simulink subsystem "MulticopterScheduler"  (R2023b)
settings: Solver=VariableStepAuto  StartTime=0.0  StopTime=10.0  RelTol=1e-3
undefined symbols (not defined in the file): CriticalTiltAngle, DiscIntNeverNeededParam, FWTrimSpeed, tilt_max, tilt_trim, uavParam, w_trim, WindDownRate
settings Model: Creator=The MathWorks, Inc.  LastModifiedBy=The MathWorks, Inc.

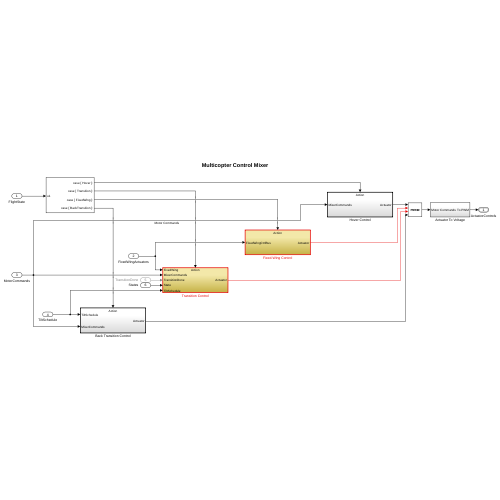
[thumbnail: Simulink's stored preview of the top-level diagram]
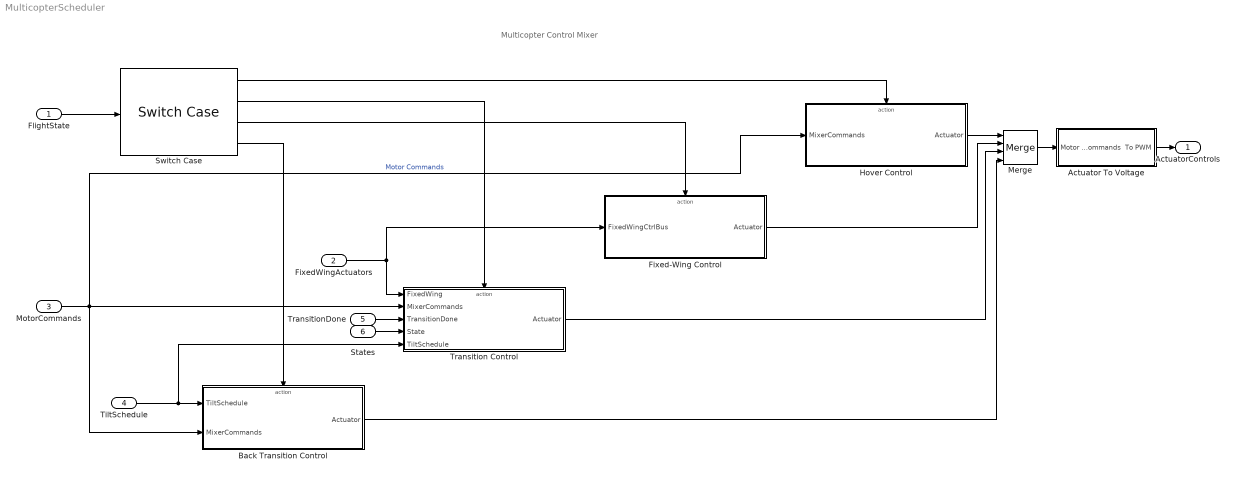
== system MulticopterScheduler ==
  note: Multicopter Control Mixer
  FlightState : Inport
  FixedWingActuators : Inport  Port=2
  MotorCommands : Inport  Port=3
  TiltSchedule : Inport  Port=4
  TransitionDone : Inport  Port=5
  States : Inport  Port=6
  Actuator To Voltage : Subsystem
  Back Transition Control : Subsystem  TreatAsAtomicUnit=on
  Fixed-Wing Control : Subsystem  TreatAsAtomicUnit=on
  Hover Control : Subsystem  TreatAsAtomicUnit=on
  Merge : Merge  Inputs=4
  Switch Case : SwitchCase  CaseConditions={flightState.Hover, flightState.Transition, flightState.FixedWing, flightState.BackTransition}  ShowDefaultCase=off
  Transition Control : Subsystem  TreatAsAtomicUnit=on
  ActuatorControls : Outport  OutDataTypeStr=Bus: RotorCntrlBus
  wires:
  Fixed-Wing Control/1(Actuator) -> Merge/2
  TiltSchedule/1 -> Transition Control/5(TiltSchedule), Back Transition Control/1(TiltSchedule)
  Switch Case/1 -> Hover Control/Action
  Merge/1 -> Actuator To Voltage/1(Motor Commands)
  FixedWingActuators/1 -> Transition Control/1(FixedWing), Fixed-Wing Control/1(FixedWingCtrlBus)
  Hover Control/1(Actuator) -> Merge/1
  Transition Control/1(Actuator) -> Merge/3
  FlightState/1 -> Switch Case/1
  TransitionDone/1 -> Transition Control/3(TransitionDone)
  States/1 -> Transition Control/4(State)
  Switch Case/4 -> Back Transition Control/Action
  Back Transition Control/1(Actuator) -> Merge/4
  MotorCommands/1 -> Back Transition Control/2(MixerCommands), Transition Control/2(MixerCommands), Hover Control/1(MixerCommands)  "Motor Commands"
  Actuator To Voltage/1(To PWM) -> ActuatorControls/1
  Switch Case/3 -> Fixed-Wing Control/Action
  Switch Case/2 -> Transition Control/Action

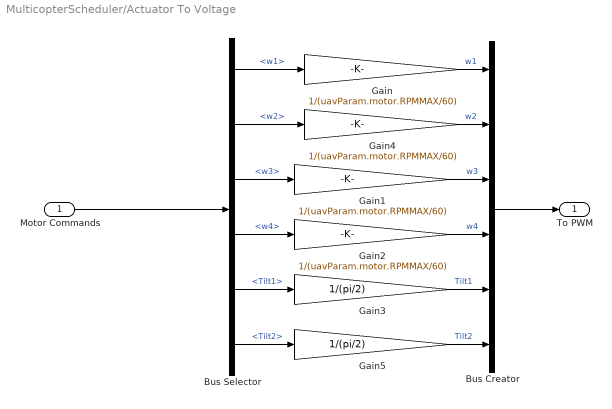
== system MulticopterScheduler/Actuator To Voltage ==
  Motor Commands : Inport
  Bus Creator : BusCreator  Inputs=6  OutDataTypeStr=Bus: RotorCntrlBus
  Bus Selector : BusSelector  OutputSignals=w1,w2,w3,w4,Tilt1,Tilt2
  Gain{,1..2,4} (4 alike) : Gain  Gain=1/(uavParam.motor.RPMMAX/60)
  Gain3 : Gain  Gain=1/(pi/2)
  Gain5 : Gain  Gain=1/(pi/2)
  To PWM : Outport
  wires:
  Bus Creator/1 -> To PWM/1
  Gain5/1 -> Bus Creator/6  "Tilt2"
  Gain3/1 -> Bus Creator/5  "Tilt1"
  Gain2/1 -> Bus Creator/4  "w4"
  Gain1/1 -> Bus Creator/3  "w3"
  Gain4/1 -> Bus Creator/2  "w2"
  Gain/1 -> Bus Creator/1  "w1"
  Bus Selector/6 -> Gain5/1  "<Tilt2>"
  Bus Selector/5 -> Gain3/1  "<Tilt1>"
  Bus Selector/4 -> Gain2/1  "<w4>"
  Bus Selector/2 -> Gain4/1  "<w2>"
  Bus Selector/3 -> Gain1/1  "<w3>"
  Bus Selector/1 -> Gain/1  "<w1>"
  Motor Commands/1 -> Bus Selector/1

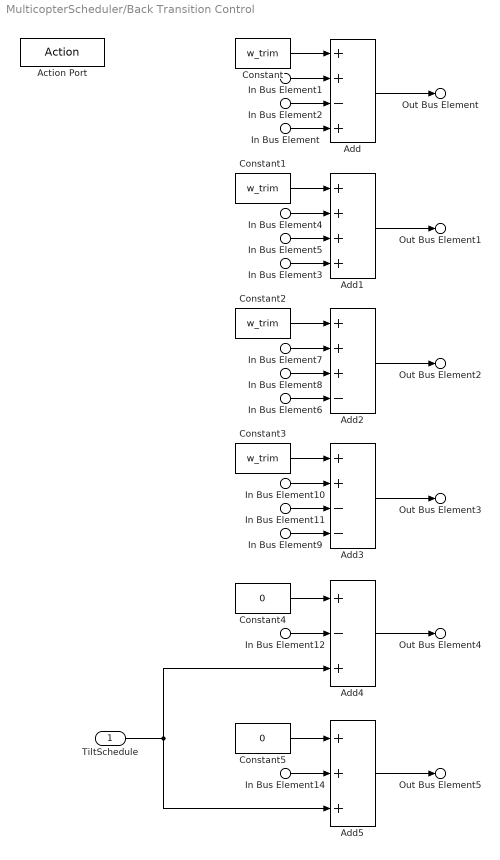
== system MulticopterScheduler/Back Transition Control ==
  TiltSchedule : Inport
  In Bus Element{,3,6,9} (4 alike) : Inport  Port=2  PortName=MixerCommands  Element=w_theta
  In Bus Element{1,4,7,10} (4 alike) : Inport  Port=2  PortName=MixerCommands  Element=w_z
  In Bus Element{2,5,8,11} (4 alike) : Inport  Port=2  PortName=MixerCommands  Element=w_phi
  In Bus Element12 : Inport  Port=2  PortName=MixerCommands  Element=l_psi
  In Bus Element14 : Inport  Port=2  PortName=MixerCommands  Element=l_psi
  Action Port : ActionPort
  Add : Sum  Inputs=++-+
  Add1 : Sum  Inputs=++++
  Add2 : Sum  Inputs=+++-
  Add3 : Sum  Inputs=++--
  Add4 : Sum  Inputs=+-+
  Add5 : Sum  Inputs=+++
  Constant{,1..3} (4 alike) : Constant  Value=w_trim
  Constant4 : Constant  Value=0
  Constant5 : Constant  Value=0
  Out Bus Element : Outport  PortName=Actuator  Element=w1
  Out Bus Element1 : Outport  PortName=Actuator  Element=w2
  Out Bus Element2 : Outport  PortName=Actuator  Element=w3
  Out Bus Element3 : Outport  PortName=Actuator  Element=w4
  Out Bus Element4 : Outport  PortName=Actuator  Element=Tilt1
  Out Bus Element5 : Outport  PortName=Actuator  Element=Tilt2
  wires:
  Add5/1 -> Out Bus Element5/1
  Add4/1 -> Out Bus Element4/1
  In Bus Element14/1 -> Add5/2
  Constant5/1 -> Add5/1
  TiltSchedule/1 -> Add5/3, Add4/3
  In Bus Element12/1 -> Add4/2
  Constant4/1 -> Add4/1
  In Bus Element7/1 -> Add2/2
  Add3/1 -> Out Bus Element3/1
  Add2/1 -> Out Bus Element2/1
  Add/1 -> Out Bus Element/1
  Constant3/1 -> Add3/1
  Constant/1 -> Add/1
  Add1/1 -> Out Bus Element1/1
  In Bus Element1/1 -> Add/2
  In Bus Element10/1 -> Add3/2
  Constant1/1 -> Add1/1
  In Bus Element6/1 -> Add2/4
  In Bus Element9/1 -> Add3/4
  Constant2/1 -> Add2/1
  In Bus Element8/1 -> Add2/3
  In Bus Element11/1 -> Add3/3
  In Bus Element/1 -> Add/4
  In Bus Element3/1 -> Add1/4
  In Bus Element5/1 -> Add1/3
  In Bus Element2/1 -> Add/3
  In Bus Element4/1 -> Add1/2

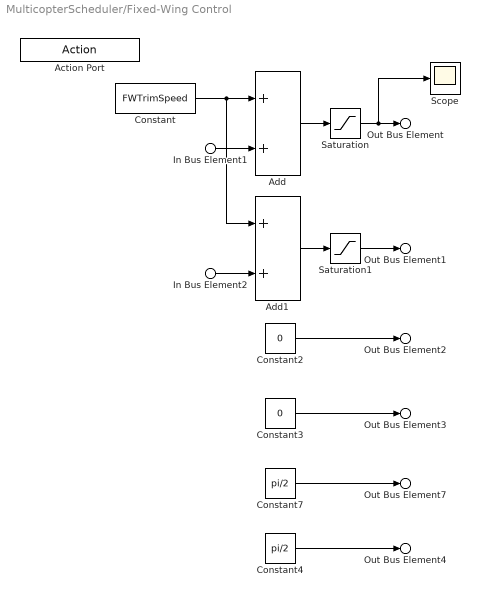
== system MulticopterScheduler/Fixed-Wing Control ==
  In Bus Element2 : Inport  PortName=FixedWingCtrlBus  Element=dT
  In Bus Element1 : Inport  PortName=FixedWingCtrlBus  Element=dT
  Action Port : ActionPort
  Add : Sum
  Add1 : Sum
  Constant : Constant  Value=FWTrimSpeed
  Constant2 : Constant  Value=0
  Constant3 : Constant  Value=0
  Constant4 : Constant  Value=pi/2
  Constant7 : Constant  Value=pi/2
  Saturation : Saturate  UpperLimit=Inf  LowerLimit=0
  Saturation1 : Saturate  UpperLimit=Inf  LowerLimit=0
  Scope : Scope
  Out Bus Element : Outport  PortName=Actuator  Element=w1
  Out Bus Element1 : Outport  PortName=Actuator  Element=w2
  Out Bus Element2 : Outport  PortName=Actuator  Element=w3
  Out Bus Element3 : Outport  PortName=Actuator  Element=w4
  Out Bus Element7 : Outport  PortName=Actuator  Element=Tilt1
  Out Bus Element4 : Outport  PortName=Actuator  Element=Tilt2
  wires:
  Constant3/1 -> Out Bus Element3/1
  Saturation1/1 -> Out Bus Element1/1
  Saturation/1 -> Out Bus Element/1, Scope/1
  In Bus Element1/1 -> Add/2
  Add/1 -> Saturation/1
  In Bus Element2/1 -> Add1/2
  Constant7/1 -> Out Bus Element7/1
  Constant/1 -> Add/1, Add1/1
  Constant2/1 -> Out Bus Element2/1
  Constant4/1 -> Out Bus Element4/1
  Add1/1 -> Saturation1/1

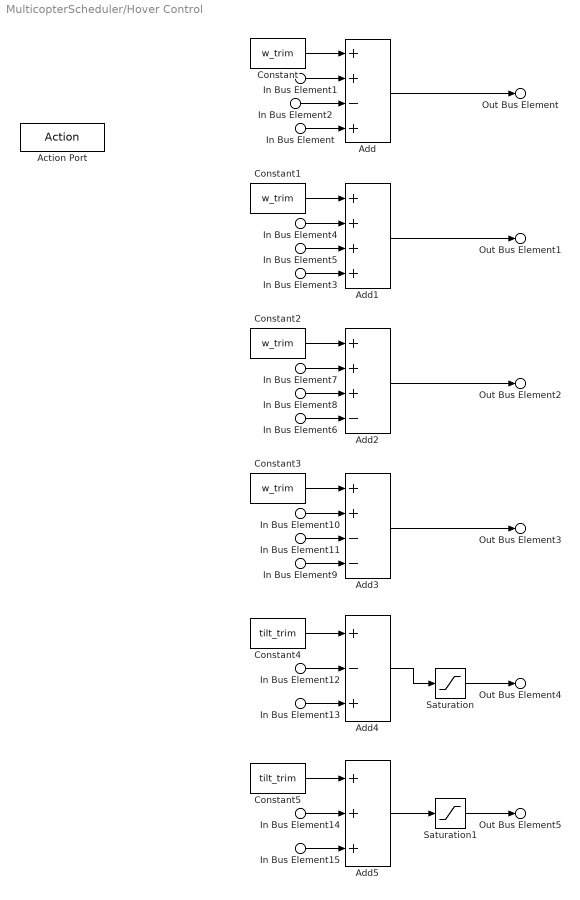
== system MulticopterScheduler/Hover Control ==
  In Bus Element{,3,6,9} (4 alike) : Inport  PortName=MixerCommands  Element=w_theta
  In Bus Element{1,4,7,10} (4 alike) : Inport  PortName=MixerCommands  Element=w_z
  In Bus Element{2,5,8,11} (4 alike) : Inport  PortName=MixerCommands  Element=w_phi
  In Bus Element12 : Inport  PortName=MixerCommands  Element=l_psi
  In Bus Element14 : Inport  PortName=MixerCommands  Element=l_psi
  In Bus Element13 : Inport  PortName=MixerCommands  Element=l_x
  In Bus Element15 : Inport  PortName=MixerCommands  Element=l_x
  Action Port : ActionPort
  Add : Sum  Inputs=++-+
  Add1 : Sum  Inputs=++++
  Add2 : Sum  Inputs=+++-
  Add3 : Sum  Inputs=++--
  Add4 : Sum  Inputs=+-+
  Add5 : Sum  Inputs=+++
  Constant{,1..3} (4 alike) : Constant  Value=w_trim
  Constant4 : Constant  Value=tilt_trim
  Constant5 : Constant  Value=tilt_trim
  Saturation : Saturate  UpperLimit=tilt_max  LowerLimit=-tilt_max
  Saturation1 : Saturate  UpperLimit=tilt_max  LowerLimit=-tilt_max
  Out Bus Element : Outport  PortName=Actuator  Element=w1
  Out Bus Element1 : Outport  PortName=Actuator  Element=w2
  Out Bus Element2 : Outport  PortName=Actuator  Element=w3
  Out Bus Element3 : Outport  PortName=Actuator  Element=w4
  Out Bus Element4 : Outport  PortName=Actuator  Element=Tilt1
  Out Bus Element5 : Outport  PortName=Actuator  Element=Tilt2
  wires:
  In Bus Element15/1 -> Add5/3
  In Bus Element14/1 -> Add5/2
  In Bus Element13/1 -> Add4/3
  In Bus Element12/1 -> Add4/2
  Saturation1/1 -> Out Bus Element5/1
  Saturation/1 -> Out Bus Element4/1
  Add3/1 -> Out Bus Element3/1
  Add2/1 -> Out Bus Element2/1
  Add1/1 -> Out Bus Element1/1
  Add/1 -> Out Bus Element/1
  In Bus Element7/1 -> Add2/2
  Add4/1 -> Saturation/1
  Constant3/1 -> Add3/1
  Constant/1 -> Add/1
  Constant4/1 -> Add4/1
  In Bus Element1/1 -> Add/2
  In Bus Element10/1 -> Add3/2
  Constant1/1 -> Add1/1
  In Bus Element6/1 -> Add2/4
  In Bus Element9/1 -> Add3/4
  Constant2/1 -> Add2/1
  In Bus Element8/1 -> Add2/3
  In Bus Element11/1 -> Add3/3
  In Bus Element/1 -> Add/4
  Add5/1 -> Saturation1/1
  In Bus Element3/1 -> Add1/4
  Constant5/1 -> Add5/1
  In Bus Element5/1 -> Add1/3
  In Bus Element2/1 -> Add/3
  In Bus Element4/1 -> Add1/2

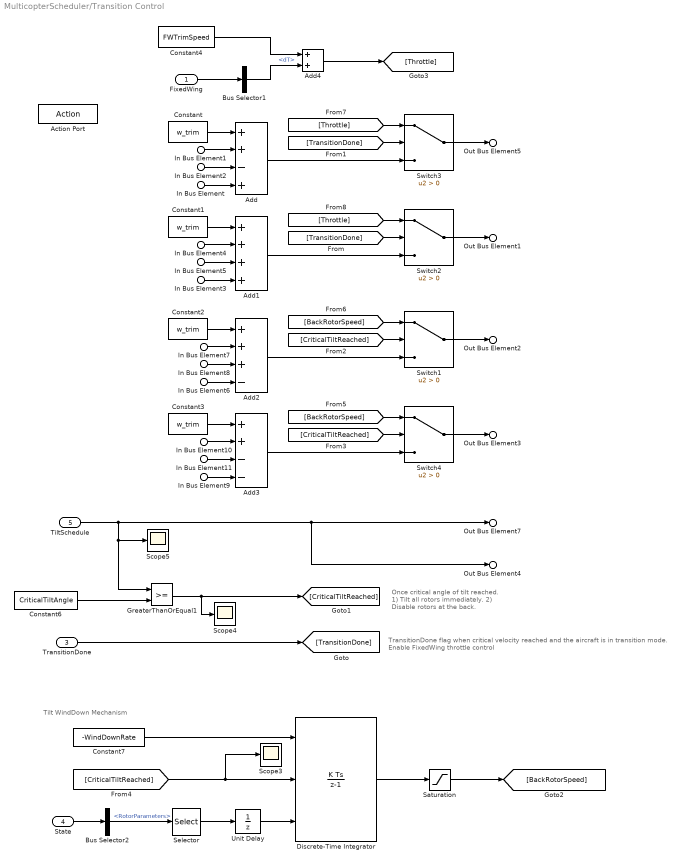
== system MulticopterScheduler/Transition Control ==
  note: TransitionDone flag when critical velocity reached and the aircraft is in transition mode.
      | Enable FixedWing throttle control
  note: Once critical angle of tilt reached.
      | 1) Tilt all rotors immediately.
      | 2) Disable rotors at the back.
  note: Tilt WindDown Mechanism
  FixedWing : Inport
  In Bus Element{,3,6,9} (4 alike) : Inport  Port=2  PortName=MixerCommands  Element=w_theta
  In Bus Element{1,4,7,10} (4 alike) : Inport  Port=2  PortName=MixerCommands  Element=w_z
  In Bus Element{2,5,8,11} (4 alike) : Inport  Port=2  PortName=MixerCommands  Element=w_phi
  TransitionDone : Inport  Port=3
  State : Inport  Port=4
  TiltSchedule : Inport  Port=5
  Action Port : ActionPort
  Add : Sum  Inputs=++-+
  Add1 : Sum  Inputs=++++
  Add2 : Sum  Inputs=+++-
  Add3 : Sum  Inputs=++--
  Add4 : Sum
  Bus Selector1 : BusSelector  OutputSignals=dT
  Bus Selector2 : BusSelector  OutputSignals=RotorParameters
  Constant{,1..3} (4 alike) : Constant  Value=w_trim
  Constant4 : Constant  Value=FWTrimSpeed
  Constant6 : Constant  Value=CriticalTiltAngle
  Constant7 : Constant  Value=-WindDownRate
  Discrete-Time Integrator : DiscreteIntegrator  ExternalReset=either  InitialConditionSource=external  SampleTime=0.005  ICPrevOutput=DiscIntNeverNeededParam  ICPrevScaledInput=DiscIntNeverNeededParam
  GreaterThanOrEqual1 : RelationalOperator  OutDataTypeStr=boolean  RndMeth=Simplest  InputSameDT=off
  Saturation : Saturate  UpperLimit=Inf  LowerLimit=0
  Scope3 : Scope
  Scope4 : Scope
  Scope5 : Scope
  Selector : Selector  InputPortWidth=6  IndexOptions=Index vector (dialog)  Indices=4  OutputSizes=1
  Switch{1..4} (4 alike) : Switch  Criteria=u2 > Threshold  SaturateOnIntegerOverflow=off  InputSameDT=off
  Unit Delay : UnitDelay  SampleTime=-1  HasFrameUpgradeWarning=on
  Out Bus Element5 : Outport  PortName=Actuator  Element=w1
  Out Bus Element1 : Outport  PortName=Actuator  Element=w2
  Out Bus Element2 : Outport  PortName=Actuator  Element=w3
  Out Bus Element3 : Outport  PortName=Actuator  Element=w4
  Out Bus Element7 : Outport  PortName=Actuator  Element=Tilt1
  Out Bus Element4 : Outport  PortName=Actuator  Element=Tilt2
  wires:
  [Throttle] -> Switch2/1
  [Throttle] -> Switch3/1
  Add4/1 -> [Throttle]
  Constant4/1 -> Add4/1
  Unit Delay/1 -> Discrete-Time Integrator/3
  State/1 -> Bus Selector2/1
  Saturation/1 -> [BackRotorSpeed]
  Discrete-Time Integrator/1 -> Saturation/1
  Selector/1 -> Unit Delay/1
  [CriticalTiltReached] -> Discrete-Time Integrator/2, Scope3/1
  Constant7/1 -> Discrete-Time Integrator/1
  Bus Selector2/1 -> Selector/1  "<RotorParameters>"
  Switch4/1 -> Out Bus Element3/1
  Switch2/1 -> Out Bus Element1/1
  Switch1/1 -> Out Bus Element2/1
  TransitionDone/1 -> [TransitionDone]
  [BackRotorSpeed] -> Switch4/1
  Add3/1 -> Switch4/3
  [CriticalTiltReached] -> Switch4/2
  [BackRotorSpeed] -> Switch1/1
  Add2/1 -> Switch1/3
  [CriticalTiltReached] -> Switch1/2
  GreaterThanOrEqual1/1 -> [CriticalTiltReached], Scope4/1
  Constant6/1 -> GreaterThanOrEqual1/2
  [TransitionDone] -> Switch3/2
  Bus Selector1/1 -> Add4/2  "<dT>"
  Switch3/1 -> Out Bus Element5/1
  FixedWing/1 -> Bus Selector1/1
  Add/1 -> Switch3/3
  [TransitionDone] -> Switch2/2
  Add1/1 -> Switch2/3
  Constant/1 -> Add/1
  In Bus Element5/1 -> Add1/3
  Constant2/1 -> Add2/1
  In Bus Element7/1 -> Add2/2
  In Bus Element4/1 -> Add1/2
  In Bus Element2/1 -> Add/3
  In Bus Element3/1 -> Add1/4
  In Bus Element11/1 -> Add3/3
  In Bus Element1/1 -> Add/2
  Constant1/1 -> Add1/1
  In Bus Element10/1 -> Add3/2
  In Bus Element/1 -> Add/4
  Constant3/1 -> Add3/1
  In Bus Element8/1 -> Add2/3
  In Bus Element6/1 -> Add2/4
  In Bus Element9/1 -> Add3/4
  TiltSchedule/1 -> Out Bus Element7/1, Out Bus Element4/1, GreaterThanOrEqual1/1, Scope5/1
